simulink model "Three_DoF_LQR"  (R2020b)
settings: Solver=VariableStepAuto  StartTime=0.0  StopTime=12  RelTol=1e-3
values from neighbouring files (symbols this model uses):
  g = 9.81    [Data_for_simulation.m]
  inertiayy = 0.048    [Data_for_simulation.m]
  K = lqr(A,B,Q,R)    [ss_3DoF_LQR.m]    (also in ss_6DoF_LQR.m)
  mass = 0.8426    [Data_for_simulation.m]
  moment_arm = 0.29    [Data_for_simulation.m]
libraries: simulink_extras x1
settings Model: Creator=tushark  LastModifiedBy=tushark
settings SolverCC: AlgebraicLoopSolver=LineSearch

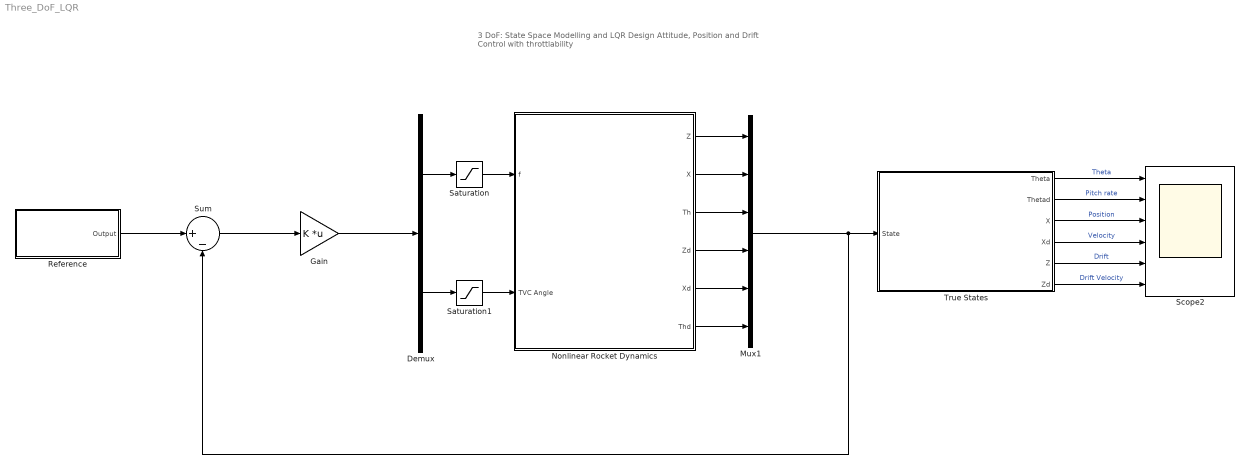
== system Three_DoF_LQR ==
  note: 3 DoF: State Space Modelling and LQR Design
      | Attitude, Position and Drift Control with throttlability
  Demux : Demux  Outputs=2
  Gain : Gain  Gain=K  Multiplication=Matrix(K*u) (u vector)
  Mux1 : Mux  Inputs=6
  Nonlinear Rocket Dynamics : Subsystem
  Reference : Subsystem
  Saturation : Saturate  UpperLimit=15  LowerLimit=0
  Saturation1 : Saturate  UpperLimit=0.174  LowerLimit=-0.174
  Scope2 : Scope  NumInputPorts=6
  Sum : Sum  Inputs=|+-
  True States : Subsystem
  wires:
  Nonlinear Rocket Dynamics/4(Zd) -> Mux1/4
  Nonlinear Rocket Dynamics/1(Z) -> Mux1/1
  Nonlinear Rocket Dynamics/3(Th) -> Mux1/3
  Demux/1 -> Saturation/1
  Nonlinear Rocket Dynamics/6(Thd) -> Mux1/6
  Nonlinear Rocket Dynamics/2(X) -> Mux1/2
  Sum/1 -> Gain/1
  Saturation/1 -> Nonlinear Rocket Dynamics/1(f)
  True States/2(Thetad) -> Scope2/2  "Pitch rate"
  True States/3(X) -> Scope2/3  "Position"
  True States/5(Z) -> Scope2/5  "Drift"
  True States/1(Theta) -> Scope2/1  "Theta"
  Nonlinear Rocket Dynamics/5(Xd) -> Mux1/5
  True States/4(Xd) -> Scope2/4  "Velocity"
  True States/6(Zd) -> Scope2/6  "Drift Velocity"
  Mux1/1 -> True States/1(State), Sum/2
  Saturation1/1 -> Nonlinear Rocket Dynamics/2(TVC Angle)
  Gain/1 -> Demux/1
  Reference/1(Output) -> Sum/1
  Demux/2 -> Saturation1/1

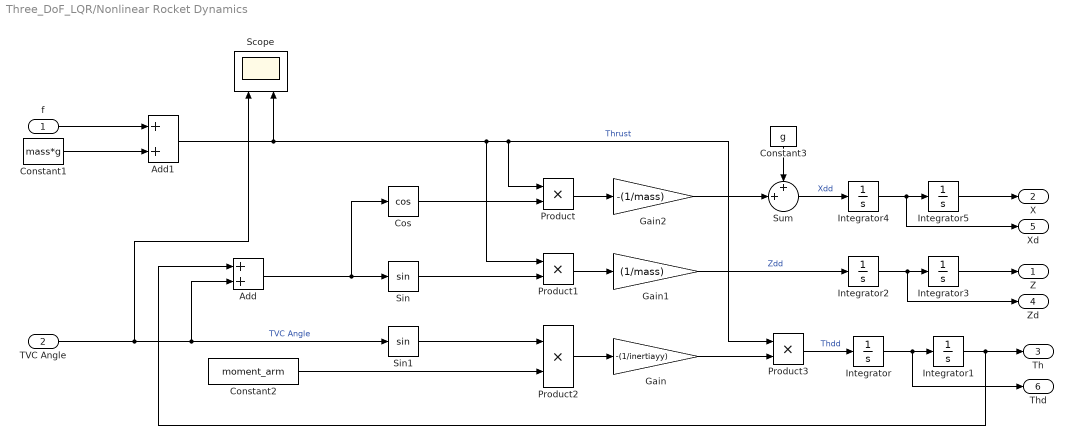
== system Three_DoF_LQR/Nonlinear Rocket Dynamics ==
  f : Inport
  TVC Angle : Inport  Port=2
  Add : Sum
  Add1 : Sum
  Constant1 : Constant  Value=mass*g
  Constant2 : Constant  Value=moment_arm
  Constant3 : Constant  Value=g
  Cos : Trigonometry  Operator=cos
  Gain : Gain  Gain=-(1/inertiayy)
  Gain1 : Gain  Gain=(1/mass)
  Gain2 : Gain  Gain=-(1/mass)
  Integrator{,2..4} (4 alike) : Integrator
  Integrator1 : Integrator  InitialCondition=0.523
  Integrator5 : Integrator  InitialCondition=30
  Product{,1..3} (4 alike) : Product
  Scope : Scope  NumInputPorts=2
  Sin : Trigonometry
  Sin1 : Trigonometry
  Sum : Sum  Inputs=++|
  Z : Outport
  X : Outport  Port=2
  Th : Outport  Port=3
  Zd : Outport  Port=4
  Xd : Outport  Port=5
  Thd : Outport  Port=6
  wires:
  Add/1 -> Cos/1, Sin/1
  Cos/1 -> Product/2
  Product/1 -> Gain2/1
  Sin/1 -> Product1/2
  f/1 -> Add1/1
  TVC Angle/1 -> Sin1/1, Add/2, Scope/1  "TVC Angle"
  Sin1/1 -> Product2/1
  Constant2/1 -> Product2/2
  Product2/1 -> Gain/1
  Integrator1/1 -> Add/1, Th/1
  Integrator4/1 -> Xd/1, Integrator5/1
  Integrator3/1 -> Z/1
  Constant1/1 -> Add1/2
  Add1/1 -> Product1/1, Product/1, Product3/1, Scope/2  "Thrust"
  Gain/1 -> Product3/2
  Product3/1 -> Integrator/1  "Thdd"
  Integrator/1 -> Thd/1, Integrator1/1
  Product1/1 -> Gain1/1
  Gain1/1 -> Integrator2/1  "Zdd"
  Integrator2/1 -> Zd/1, Integrator3/1
  Integrator5/1 -> X/1
  Gain2/1 -> Sum/2
  Sum/1 -> Integrator4/1  "Xdd"
  Constant3/1 -> Sum/1

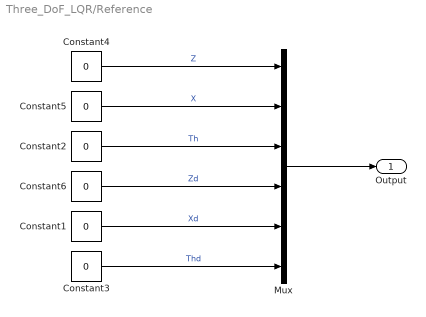
== system Three_DoF_LQR/Reference ==
  Constant{1..6} (6 alike) : Constant  Value=0
  Mux : Mux  Inputs=6
  Output : Outport
  wires:
  Constant1/1 -> Mux/5  "Xd"
  Constant3/1 -> Mux/6  "Thd"
  Constant2/1 -> Mux/3  "Th"
  Constant6/1 -> Mux/4  "Zd"
  Constant4/1 -> Mux/1  "Z"
  Constant5/1 -> Mux/2  "X"
  Mux/1 -> Output/1

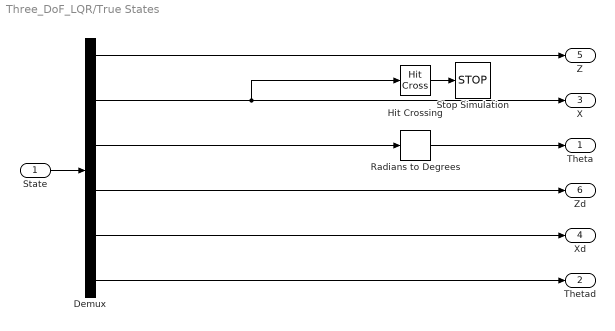
== system Three_DoF_LQR/True States ==
  State : Inport
  Demux : Demux  Outputs=6
  Hit Crossing : HitCross  HitCrossingDirection=falling
  Radians to Degrees : simulink_extras/Transformations/Radians to Degrees
  Stop Simulation : Stop
  Theta : Outport
  Thetad : Outport  Port=2
  X : Outport  Port=3
  Xd : Outport  Port=4
  Z : Outport  Port=5
  Zd : Outport  Port=6
  wires:
  Demux/5 -> Xd/1
  Radians to Degrees/1 -> Theta/1
  Demux/3 -> Radians to Degrees/1
  Demux/6 -> Thetad/1
  Demux/2 -> Hit Crossing/1, X/1
  Demux/4 -> Zd/1
  Demux/1 -> Z/1
  Hit Crossing/1 -> Stop Simulation/1
  State/1 -> Demux/1
